simulink model "URBANWAY"  (R2021a)
settings: Solver=FixedStepAuto  StartTime=0.0  StopTime=1500  FixedStep=0.5  RelTol=1e-3
undefined symbols (not defined in the file): a_braking, BatCap, curv, d, eta, gradient, i, m, me, P_aux, P_engine, rpm_em, SOC0, SOCl, SOCu, speed_limits, speed_limits_positions, stops_positions, T_em, wheel_radius
libraries: simulink x12, simulink_extras x1
settings Model: PacingRate=4  Creator=feder  LastModifiedBy=feder
settings SolverCC: ZeroCrossAlgorithm=Adaptive
settings DebuggingCC: IgnoredZcDiagnostic=none  UnderSpecifiedDimensionMsg=warning

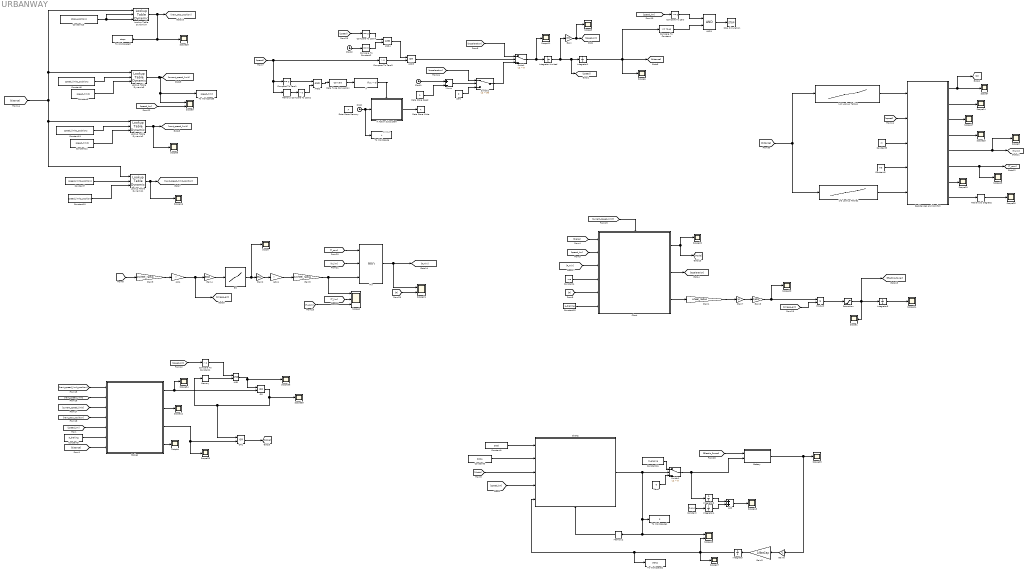
== system URBANWAY ==
  note: simout
  1-D Lookup Table1 : Lookup_n-D  NumberOfTableDimensions=1  BreakpointsForDimension1=d  Table=curv  InternalRulePriority=Speed  RndMeth=Simplest  InputSameDT=on
  1-D Lookup Table2 : Lookup_n-D  NumberOfTableDimensions=1  BreakpointsForDimension1=d  Table=gradient  InternalRulePriority=Speed  RndMeth=Simplest  InputSameDT=on
  AND{,1..2,4} (4 alike) : Logic  AllPortsSameDT=off  OutDataTypeStr=boolean
  AND3 : Logic  Operator=OR  AllPortsSameDT=off  OutDataTypeStr=boolean
  Add : Sum
  Battery : MATLAB Function  TreatAsAtomicUnit=on
  Brakes : MATLAB Function  TreatAsAtomicUnit=on
  Chart : Stateflow chart  TreatAsAtomicUnit=on
      settings: PortSchema="{\"entries\":[{\"content\":{\"sides\":[{\"content\":{\"connectorIds\":[\"In2\",\"In3\",\"In7\",\"In4\",\"In5\",\"In6\"]},\"type\":\"ConnectorPlacement.EquallySpacedRectSide\",\"uuid\":\"078ca5c4-d963-4c25-bdb2-9f3ae7ec6874\"},{\"content\":{\"connectorIds\":[\"Out1\",\"Out2\",\"Out3\"],\"side\":\"RIGHT\"},\"type\":\"ConnectorPlacement.EquallySpacedRectSide\",\"uuid\":\"67d936b2-2c10-44c4-9d07-6b02e6932369\"},{\"content\":{\"connectorIds\":[\"In1\"],\"side\":\"TOP\"},\"type\":\"ConnectorPlacement.EquallySpacedRectSide\",\"uuid\":\"e07d9aa8-906c-4eaa-aced-e56d89c71485\"}]},\"type\":\"ConnectorPlacement.EquallySpacedConnector\",\"uuid\":\"666db62f-681a-4c26-b64e-f559fb384b7b\"}],\"packageUris\":[\"http://schema.mathworks.com/mf0/Connector/R2020b\"],\"version\":\"1.0\"}"
  Chart2 : Stateflow chart  TreatAsAtomicUnit=on
      settings: PortSchema="{\"entries\":[{\"content\":{\"sides\":[{\"content\":{\"connectorIds\":[\"In3\",\"In1\",\"In4\",\"In5\",\"In2\"]},\"type\":\"ConnectorPlacement.EquallySpacedRectSide\",\"uuid\":\"621613b0-231b-4daf-be7e-6dcd3d0c6566\"},{\"content\":{\"connectorIds\":[\"Out1\"],\"side\":\"RIGHT\"},\"type\":\"ConnectorPlacement.EquallySpacedRectSide\",\"uuid\":\"af18cd7e-6c98-4eea-b647-f0f04560d8c6\"},{\"content\":{\"connectorIds\":[],\"side\":\"TOP\"},\"type\":\"ConnectorPlacement.EquallySpacedRectSide\",\"uuid\":\"58f19e9d-2d8b-4d3d-8d3c-b9c66059b3f7\"},{\"content\":{\"connectorIds\":[\"In6\"],\"side\":\"BOTTOM\"},\"type\":\"ConnectorPlacement.EquallySpacedRectSide\",\"uuid\":\"ce09c1ac-99c2-4b05-ab8b-8cad14ac8309\"}]},\"type\":\"ConnectorPlacement.EquallySpacedConnector\",\"uuid\":\"0dc2274d-f112-48bf-9fd5-23ea08679248\"}],\"packageUris\":[\"http://schema.mathworks.com/mf0/Connector/R2020b\"],\"version\":\"1.0\"}"
  Clock : Clock
  Clock1 : Clock
  Clock2 : Clock
  Compare To Constant : simulink/Logic and Bit Operations/Compare To Constant  relop=>=  const=7240  OutDataTypeStr=boolean
  Compare To Constant1 : simulink/Logic and Bit Operations/Compare To Constant  relop=>  const=0  OutDataTypeStr=boolean
  Compare To Constant2 : simulink/Logic and Bit Operations/Compare To Constant  relop===  const=0  OutDataTypeStr=boolean
  Compare To Zero : simulink/Logic and Bit Operations/Compare To Zero  relop=<=  OutDataTypeStr=boolean
  Compare To Zero1 : simulink/Logic and Bit Operations/Compare To Zero  relop===  OutDataTypeStr=boolean
  Compare To Zero2 : simulink/Logic and Bit Operations/Compare To Zero  relop=>  OutDataTypeStr=boolean
  Compare To Zero3 : simulink/Logic and Bit Operations/Compare To Zero  relop=>  OutDataTypeStr=boolean
  Compare To Zero4 : simulink/Logic and Bit Operations/Compare To Zero  relop===  OutDataTypeStr=boolean
  Constant : Constant  Value=P_aux
  Constant1 : Constant  Value=SOCl
  Constant{7..8,10..11} (4 alike) : Constant  Value=speed_limits_positions
  Constant12 : Constant  Value=speed_limits
  Constant13 : Constant  Value=stops_positions
  Constant15 : Constant  Value=a_braking
  Constant16 : Constant  Value=P_engine
  Constant2 : Constant  Value=me
  Constant3 : Constant  Value=m
  Constant4 : Constant  Value=me
  Constant5 : Constant  Value=a_braking
  Constant6 : Constant  Value=SOCu
  Constant9 : Constant  Value=speed_limits
  Data Store Read : DataStoreRead  IndexOptions=Index vector (dialog)  Indices=1  OutputSizes=1
  Data Store Write : DataStoreWrite  IndexOptions=Index vector (dialog)  Indices=1  OutputSizes=1
  Data Store Memory : DataStoreMemory  ReadBeforeWriteMsg=warning  WriteAfterWriteMsg=warning  WriteAfterReadMsg=warning  ShowAdditionalParam=off
  Data Type Conversion : DataTypeConversion
  EM : Lookup_n-D  NumberOfTableDimensions=1  BreakpointsForDimension1=rpm_em  Table=T_em  InternalRulePriority=Speed  RndMeth=Simplest  InputSameDT=on
  Gain : Gain  Gain=3.6
  Gain1 : Gain  Gain=wheel_radius
  Gain2 : Gain  Gain=eta
  Gain3 : Gain  Gain=1/BatCap
  Gain4 : Gain  Gain=30/pi
  Gain5 : Gain  Gain=1/wheel_radius
  Gain6 : Gain  Gain=-1
  Gain7 : Gain  Gain=1/i
  Gain8 : Gain  Gain=1/eta
  Gain9 : Gain  Gain=1/wheel_radius
  If : If  ShowElse=off
  If Action Subsystem : Subsystem  TreatAsAtomicUnit=on
  Integrator : Integrator  InitialCondition=SOC0
  Integrator Limited : Integrator  LimitOutput=on  UpperSaturationLimit=1000  LowerSaturationLimit=0
  Integrator{1..4} (4 alike) : Integrator
  Lookup Table Dynamic1 : simulink/Lookup Tables/Lookup Table Dynamic  LookUpMeth=Use Input Above  OutDataType=fixdt('double')  OutScaling=[]  OutputDataTypeScalingMode=Specify via dialog  OutDataTypeStr=double  DoSatur=off
  Lookup Table Dynamic2 : simulink/Lookup Tables/Lookup Table Dynamic  LookUpMeth=Use Input Above  OutDataType=fixdt('double')  OutScaling=[]  OutputDataTypeScalingMode=Specify via dialog  OutDataTypeStr=double  DoSatur=off
  Lookup Table Dynamic3 : simulink/Lookup Tables/Lookup Table Dynamic  LookUpMeth=Use Input Below  OutDataType=fixdt('double')  OutScaling=[]  OutputDataTypeScalingMode=Specify via dialog  OutDataTypeStr=double  DoSatur=off
  Lookup Table Dynamic4 : simulink/Lookup Tables/Lookup Table Dynamic  LookUpMeth=Use Input Above  OutDataType=fixdt('double')  OutScaling=[]  OutputDataTypeScalingMode=Specify via dialog  OutDataTypeStr=double  DoSatur=off
  Memory : Memory
  Memory1 : Memory
  Memory2 : Memory  InitialCondition=1
  Min : MinMax  Inputs=3
  Minus : Sum  Inputs=+-
  OR : Logic  Operator=OR  AllPortsSameDT=off  OutDataTypeStr=boolean
  OR1 : Logic  Operator=OR  AllPortsSameDT=off  OutDataTypeStr=boolean
  Product : Product
  Radians to Degrees : simulink_extras/Transformations/Radians to Degrees
  Resistances and Comfort : MATLAB Function  TreatAsAtomicUnit=on
  Saturation : Saturate  UpperLimit=500e+03  LowerLimit=0.3*(-160e+03)
  Scope{,1,3..8,11..14,16..20,22..28,33..36} (28 alike) : Scope
  Scope15 : Scope  NumInputPorts=2
  Scope2 : Scope  NumInputPorts=3
  Scope21 : Scope  NumInputPorts=2
  Scope9 : Scope  NumInputPorts=2
  Stop Simulation : Stop
  Switch : Switch  Criteria=u2 > Threshold
  Switch1 : Switch  Criteria=u2 > Threshold
  Switch2 : Switch  Criteria=u2 > Threshold  Threshold=30
  To Workspace : ToWorkspace  VariableName=t  SampleTime=-1
  To Workspace1 : ToWorkspace  VariableName=S  SampleTime=-1
  To Workspace2 : ToWorkspace  VariableName=SOC1  SampleTime=-1
  To Workspace3 : ToWorkspace  VariableName=stops  SampleTime=-1
  To Workspace5 : ToWorkspace  VariableName=speed_limit  SaveFormat=Timeseries  SampleTime=-1
  Zero : Constant  Value=0  OutDataTypeStr=Inherit: Inherit via back propagation
  Zero1 : Constant  Value=0  OutDataTypeStr=Inherit: Inherit via back propagation
  ratio : Gain  Gain=i
  ratio1 : Gain  Gain=i
  wires:
  Switch/1 -> Scope11/1, Integrator Limited/1
  Integrator1/1 -> Compare To Constant/1, [distance], Scope6/1
  Constant5/1 -> Brakes/6(a_braking)
  [distance] -> Brakes/7(s)
  [speed_km] -> Brakes/5(vkm)
  Gain/1 -> Scope5/1, [speed_km]
  1-D Lookup Table1/1 -> Resistances and Comfort/1(curv)
  1-D Lookup Table2/1 -> Resistances and Comfort/5(gradient)
  Resistances and Comfort/1(R) -> Scope7/1, [R]
  [speed_km] -> Chart/3(speed_km)
  [brake] -> Chart/2(Brake)
  [R] -> Chart/5(R)
  Constant4/1 -> Chart/4(me)
  Chart/1(Mode) -> Scope22/1, [Mode]
  Chart/2(a) -> [acceleration]
  [speed] -> Resistances and Comfort/2(v)
  Constant3/1 -> Resistances and Comfort/3(m)
  Resistances and Comfort/3(Ri) -> Scope17/1
  Resistances and Comfort/4(Ra) -> Scope25/1
  Constant11/1 -> Lookup Table Dynamic2/2
  Constant12/1 -> Lookup Table Dynamic2/3
  Constant7/1 -> Lookup Table Dynamic1/2
  Lookup Table Dynamic1/1 -> Scope16/1, [next_speed_limit_position]
  Constant10/1 -> Lookup Table Dynamic1/3
  Lookup Table Dynamic2/1 -> Scope8/1, [next_speed_limit]
  Lookup Table Dynamic3/1 -> Scope9/1, To Workspace5/1, [current_speed_limit]
  Constant8/1 -> Lookup Table Dynamic3/2
  Constant9/1 -> Lookup Table Dynamic3/3
  [next_speed_limit_position] -> Brakes/1(next_speed_limit_position)
  [next_speed_limit] -> Brakes/2(next_speed_limit)
  [current_speed_limit] -> Brakes/3(current_speed_limit)
  Constant13/1 -> Lookup Table Dynamic4/3, Lookup Table Dynamic4/2
  Lookup Table Dynamic4/1 -> Scope28/1, To Workspace3/1, [next_stop_position]
  [next_stop_position] -> Brakes/4(next_stop_position)
  [current_speed_limit] -> Chart/1(current_speed_limit)
  Constant15/1 -> Chart/6(a_braking)
  Brakes/2(B2) -> Scope12/1
  [speed_km] -> Compare To Constant1/1
  AND/1 -> Scope36/1, OR/1
  OR/1 -> Memory/1, OR1/1, Scope35/1
  Memory/1 -> AND/2
  [distance] -> Lookup Table Dynamic1/1, Lookup Table Dynamic2/1, Lookup Table Dynamic4/1, Lookup Table Dynamic3/1
  Compare To Constant1/1 -> AND/1
  OR1/1 -> [brake]
  Brakes/1(Brake2) -> Scope34/1, OR/2
  Brakes/3(Brake1) -> Scope33/1, OR1/2
  [speed_km] -> Compare To Zero/1
  Compare To Constant/1 -> AND1/2
  Compare To Zero/1 -> AND1/1
  AND1/1 -> Stop Simulation/1
  [acceleration] -> Switch/1
  Resistances and Comfort/7(a_lat) -> Scope19/1
  Resistances and Comfort/6(T_com) -> Scope13/1, [T_com]
  Constant2/1 -> Resistances and Comfort/4(me)
  Resistances and Comfort/5(T_lim) -> Scope3/1, [T_lim]
  [T_com] -> Min/1
  [T_lim] -> Min/2
  EM/1 -> Scope/1, Gain2/1
  Constant1/1 -> Chart2/3(SOCl)
  Chart/3(F) -> Gain1/1
  Resistances and Comfort/2(Rv) -> Scope14/1
  [R] -> Scope21/2
  Integrator Limited/1 -> [speed], Integrator1/1, Gain/1
  Switch2/1 -> Switch/3
  If Action Subsystem/1(Out1) -> Data Store Write/1
  Data Store Read/1 -> Minus/2
  Clock1/1 -> Minus/1
  Zero/1 -> Switch2/3
  Data Type Conversion/1 -> If/1
  Clock/1 -> To Workspace/1, If Action Subsystem/1(In1)
  Compare To Zero1/1 -> AND2/1
  Minus/1 -> Switch2/2
  [acceleration] -> Switch2/1
  Memory1/1 -> Compare To Zero2/1
  AND2/1 -> Data Type Conversion/1
  [T_com] -> Scope2/3
  [speed] -> Gain9/1
  Gain9/1 -> ratio/1
  Constant6/1 -> Chart2/1(SOCu)
  Chart2/1(S) -> Scope15/1, Memory2/1, To Workspace1/1, Switch1/2
  Constant16/1 -> Switch1/1
  Zero1/1 -> Switch1/3
  Switch1/1 -> Battery/2(P_gen), Integrator2/1
  Product/1 -> Saturation/1
  [omega_em] -> Product/2
  Gain4/1 -> EM/1
  ratio/1 -> Gain4/1, [omega_em]
  Gain1/1 -> Gain7/1
  Gain5/1 -> Min/3, Scope2/1
  Saturation/1 -> Scope1/1, [Electric_Power], Integrator3/1
  [speed_km] -> Scope9/2
  Integrator3/1 -> Scope24/1
  Brakes/4(B1) -> Scope4/1
  Resistances and Comfort/8(theta) -> Radians to Degrees/1
  Radians to Degrees/1 -> Scope26/1
  Integrator/1 -> Scope27/1, To Workspace2/1, Chart2/2(SOC), Scope15/2
  Battery/1(Ibat1) -> Scope23/1, Gain6/1
  [speed_km] -> Chart2/5(speed_km)
  [Mode] -> Chart2/4(Mode)
  Memory2/1 -> Chart2/6(S1)
  Gain6/1 -> Gain3/1
  Gain3/1 -> Integrator/1
  [T_lim] -> Scope2/2
  Min/1 -> [F_min], Scope21/1
  [F_min] -> Chart/7(F_required)
  [Electric_Power] -> Battery/1(P_em)
  If/1 -> If Action Subsystem/Action
  Compare To Zero2/1 -> AND2/2
  [speed] -> Memory1/1, Compare To Zero1/1, Compare To Zero3/1
  Clock2/1 -> Compare To Constant2/1
  Compare To Zero3/1 -> AND3/2
  AND3/1 -> Switch/2
  [speed] -> Compare To Zero4/1
  Compare To Constant2/1 -> AND4/2
  Compare To Zero4/1 -> AND4/1
  AND4/1 -> AND3/1
  Constant/1 -> Integrator4/1
  Integrator4/1 -> Add/2
  Integrator2/1 -> Add/1
  Add/1 -> Scope18/1
  [distance] -> 1-D Lookup Table1/1, 1-D Lookup Table2/1
  Gain7/1 -> Gain8/1
  Gain2/1 -> ratio1/1
  ratio1/1 -> Gain5/1
  Gain8/1 -> Scope20/1, Product/1

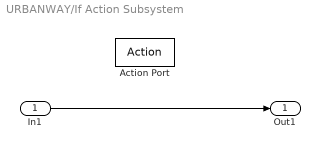
== system URBANWAY/If Action Subsystem ==
  In1 : Inport
  Action Port : ActionPort  ActionPortLabel=if(u1 > 0)
  Out1 : Outport
  wires:
  In1/1 -> Out1/1

== matlab function URBANWAY/Brakes ==
  data: Brake2 output; B2 output; Brake1 output; next_speed_limit_position input; next_speed_limit input; current_speed_limit input; next_stop_position input; vkm input; a_braking input; s input; B1 output
function [Brake2, B2, Brake1, B1] = fcn(next_speed_limit_position, next_speed_limit, current_speed_limit, next_stop_position, vkm, a_braking, s)

v=vkm/3.6;
Brake1=false;
Brake2=false;
B1=0;
if vkm > current_speed_limit
    
    Brake1=true;
end


if next_speed_limit <  vkm
    
    dbr = (v^2-(next_speed_limit/3.6)^2)/(2*a_braking);
    B1= next_speed_limit_position-(dbr+s);


    if B1<=0
        
        Brake1 = true;
    end
    
end

dbr = (v^2)/(2*a_braking);
B2=next_stop_position-(dbr+s);

if B2<0
    
    Brake2 = true;
    
end

% Brake=Brake1 | Brake2;

end

== stateflow chart URBANWAY/Chart2 ==
  state ICE_ON
    S=1;
  state REGENERATIVE_BRAKING
    S=0;
  state ICE_OFF
    S=0;
  state HOLD
    S=S1;
  ICE_OFF -> ICE_ON [order 1] : [SOC <=  SOCl && Mode~=3]
  ICE_ON -> HOLD [order 3] : [SOC < SOCu && SOC>SOCl && Mode ~=3]
  HOLD -> ICE_ON [order 2] : [SOC <=  SOCl && Mode~=3]
  ICE_ON -> ICE_OFF [order 2] : [(SOC >=SOCu || (speed_km<20 && SOC >SOCl)) && Mode~=3]
  ICE_ON -> REGENERATIVE_BRAKING [order 1] : [Mode==3]
  REGENERATIVE_BRAKING -> ICE_ON [order 2] : [ SOC<=SOCl && Mode~=3]
  (default) -> ICE_OFF
  ICE_OFF -> REGENERATIVE_BRAKING [order 3] : [Mode==3]
  REGENERATIVE_BRAKING -> ICE_OFF [order 3] : [(SOC >= SOCu || (speed_km<20 && SOC >SOCl)) && Mode~=3]
  HOLD -> REGENERATIVE_BRAKING [order 1] : [Mode==3]
  REGENERATIVE_BRAKING -> HOLD [order 1] : [SOC < SOCu && SOC>SOCl && Mode ~=3]
  ICE_OFF -> HOLD [order 2] : [SOC < SOCu && SOC>SOCl && Mode ~=3]
  HOLD -> ICE_OFF [order 3] : [(SOC >= SOCu || (speed_km<20 && SOC >SOCl)) && Mode~=3 && S1==1]
  data: SOCu input; SOC input; SOCl input; Mode input; speed_km input; S output; S1 input

== matlab function URBANWAY/Resistances and Comfort ==
  data: curv input; v input; m input; me input; R output; Rv output; gradient input; Ri output; Ra output; T_lim output; T_com output; a_lat output; theta output
function [R, Rv, Ri, Ra, T_lim , T_com, a_lat, theta] = fcn(curv, v, m, me, gradient)


a_com=0.8;
A_front=2.5*2.393;
C_d=0.33;

Ra=1/2*1.225*C_d*A_front*v^2;

Ri=m*9.81*sin(deg2rad(gradient));

Rv=m*9.81*0.014*cos(deg2rad(gradient));

a_lat=v^2*curv;

h=0.5;
B=2.5;
H=2.893;
g=9.81;
M=26400;
ky=320e+03;
kr=400; %Nm/rad

theta=M*H*a_lat/(ky*B^2+2*kr-M*g*H);
%alpha=1/8;
%theta=(B/H)*(1+alpha)-a_lat/g*(1+(h/H)*(2+alpha));


T_lim=0.8*(m*9.18*cos(deg2rad(gradient))+m*a_lat);
R = Ra + Ri + Rv;

T_com=me*a_com+R;

end

== stateflow chart URBANWAY/Chart ==
  state STOP
    Mode=4;
    F=0;
    a=(F_required-R)/me;
  state BRAKING
    Mode=3;
    a=-a_braking;
    F=me*a+R;
  state TRACTION
    Mode=1;
    F=F_required;
    a=(F-R)/me;
  state FREE_RUNNING
    if R<0
    Mode=3;
    else
    Mode=2;
    end
    F=R;
    a=0;
  (default) -> STOP
  BRAKING -> STOP [order 2] : [speed_km<=0]
  STOP -> TRACTION : [speed_km>0]
  TRACTION -> BRAKING [order 1] : [Brake==true]
  BRAKING -> TRACTION [order 1] : [Brake==false && speed_km<current_speed_limit -2 && speed_km>0 ]
  FREE_RUNNING -> BRAKING [order 1] : [Brake==true || Mode==3]
  BRAKING -> FREE_RUNNING [order 3] : [Brake==false && speed_km>current_speed_limit -2 ]
  FREE_RUNNING -> TRACTION [order 2] : [speed_km<current_speed_limit -2 && Brake==false]
  TRACTION -> FREE_RUNNING [order 2] : [speed_km>current_speed_limit -2  && Brake==false]
  data: current_speed_limit input; Brake input; speed_km input; Mode output; me input; a output; R input; a_braking input; F_required input; F output

== matlab function URBANWAY/Battery ==
  data: Ibat1 output; P_em input; P_gen input
function Ibat1  = fcn(P_em, P_gen)

V0=635;
Q=11e+03;%Wh
R=0.17; %Ohm

if P_em<0
    P_em=0.3*P_em;
end

Ibat1=(V0-sqrt(V0^2-4*R*(P_em-P_gen)))/(2*R);

end
